simulink model "Week3_LOC4_deel1_v2_1"  (R2021b)
settings: Solver=FixedStepDiscrete  StartTime=0.0  StopTime=inf  RelTol=1e-3
libraries: arduinolib x5
settings Model: FPTRunName=Active  ExtModeTrigDuration=2  Creator=889450  LastModifiedBy=Jeedella
settings SolverCC: AlgebraicLoopSolver=TrustRegion
settings DataIOCC: LimitDataPoints=on  SaveFormat=Array
settings OptimizationCC: ExpressionDepthLimit=2147483647  LifeSpan=Inf  MaxStackSize=64
settings DebuggingCC: UnderspecifiedInitializationDetection=Classic  MergeDetectMultiDrivingBlocksExec=none  FcnCallInpInsideContextMsg=warning  AllowSymbolicDim=off  StateNameClashWarn=warning  SFUnexpectedBacktrackingDiag=warning  SFNoUnconditionalDefaultTransitionDiag=warning  SFExecutionAtInitializationDiag=none  SFMachineParentedDataDiag=warning  ArithmeticOperatorsInVariantConditions=warning
settings HardwareCC: ProdBitPerInt=16  ProdBitPerPointer=16  ProdBitPerSizeT=16  ProdBitPerPtrDiffT=16  ProdLargestAtomicFloat=None  ProdWordSize=8  ProdHWDeviceType=Atmel->AVR
settings ModelReferenceCC: PropagateSignalLabelsOutOfModel=off
settings SFSimCC: SimUseLocalCustomCode=off  CustomCodeUndefinedFunction=UseInterfaceOnly
settings RTWCC: Description=Embedded Coder  SystemTargetFile=ert.tlc  HardwareBoard=Arduino Uno  TemplateMakefile=ert_default_tmf  GenerateReport=on  RTWVerbose=off  RTWUseLocalCustomCode=off  Toolchain=Arduino AVR  BuildConfiguration=Faster Runs  LaunchReport=on
settings CodeAppCC: ForceParamTrailComments=on  OperatorAnnotations=on  StateflowObjectComments=on  MATLABSourceComments=on
settings ERTTargetCC: MultiwordLength=2048  ERTCustomFileBanners=off  SupportContinuousTime=on  SupportNonInlinedSFcns=on  RemoveResetFunc=off  SupportVariableSizeSignals=on  ModelStepFunctionPrototypeControlCompliant=off  ExtModeStaticAllocSize=250
settings ConfigComp: CovMetricSettings=dw  CovSaveCumulativeToWorkspaceVar=on  CovSaveSingleToWorkspaceVar=on  CovExternalEMLEnable=off  CovSFcnEnable=off

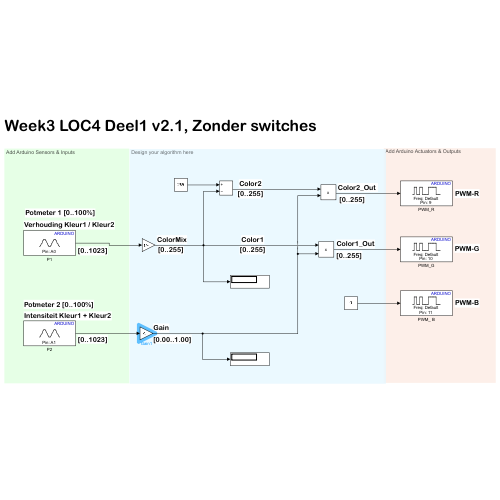
[thumbnail: Simulink's stored preview of the top-level diagram]
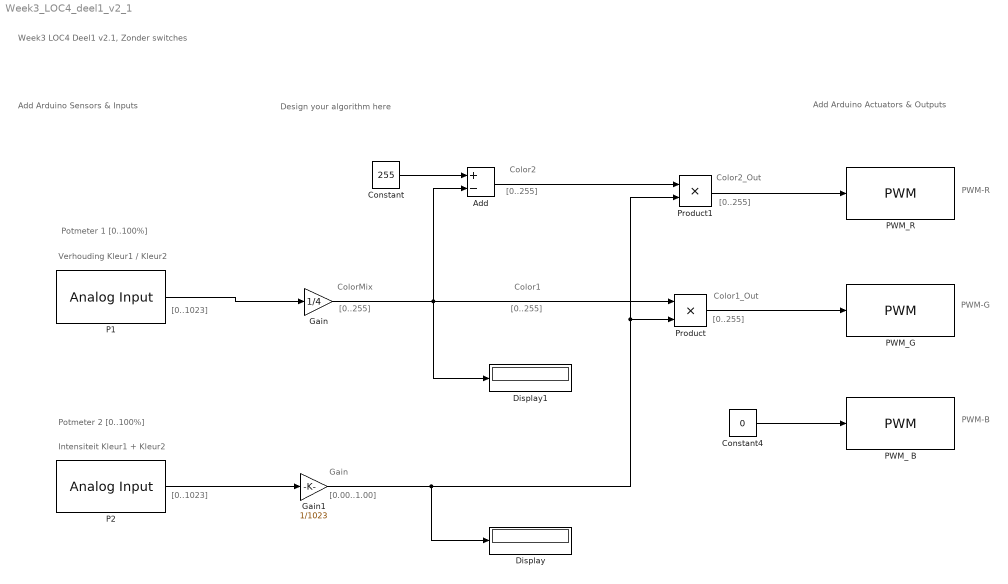
== system Week3_LOC4_deel1_v2_1 ==
  note: Week3 LOC4 Deel1 v2.1, Zonder switches
  note: Potmeter 1 [0..100%]
  note: Potmeter 2 [0..100%]
  note: Verhouding Kleur1 / Kleur2
  note: Intensiteit Kleur1 + Kleur2
  note: [0..1023]
  note: [0..1023]
  note: [0..255]
  note: [0.00..1.00]
  note: Gain
  note: [0..255]
  note: Color1_Out
  note: Color2_Out
  note: PWM-R
  note: PWM-G
  note: PWM-B
  note: Add Arduino Sensors & Inputs
  note: Add Arduino Actuators & Outputs
  note: Design your algorithm here
  note: ColorMix
  note: Color1
  note: [0..255]
  note: [0..255]
  note: Color2
  note: [0..255]
  Add : Sum  Inputs=+-
  Constant : Constant  Value=255  SampleTime=-1
  Constant4 : Constant  Value=0  SampleTime=-1
  Display : Display
  Display1 : Display
  Gain : Gain  Gain=1/4
  Gain1 : Gain  Gain=1/1023
  P1 : arduinolib/Analog Input  pinNumber=0  ReadResultsOnly=off  ConversionTriggerSource=Software  ExternalTriggerType=uint32( 0 )  OutputDataType=uint16  EnableConversionCompleteNotify=off  EnableOuputStatus=off  SampleTime=-1  blockPlatform=arduino
  P2 : arduinolib/Analog Input  pinNumber=1  ReadResultsOnly=off  ConversionTriggerSource=Software  ExternalTriggerType=uint32( 0 )  OutputDataType=uint16  EnableConversionCompleteNotify=off  EnableOuputStatus=off  SampleTime=-1  blockPlatform=arduino
  PWM_ B : arduinolib/PWM  pinNumber=11  frequencyType=Default  desiredFrequency=490.2  achievableFrequency=490.2
  PWM_G : arduinolib/PWM  pinNumber=10  frequencyType=Default  desiredFrequency=490.2  achievableFrequency=490.2
  PWM_R : arduinolib/PWM  pinNumber=9  frequencyType=Default  desiredFrequency=490.2  achievableFrequency=490.2
  Product : Product
  Product1 : Product
  wires:
  P1/1 -> Gain/1
  Gain/1 -> Add/2, Product/1, Display1/1
  Add/1 -> Product1/1
  Constant/1 -> Add/1
  P2/1 -> Gain1/1
  Gain1/1 -> Product1/2, Product/2, Display/1
  Product/1 -> PWM_G/1
  Constant4/1 -> PWM_ B/1
  Product1/1 -> PWM_R/1
